simulink model "ACC_Model"  (Simulink 7.6)
settings: Solver=ode5  StartTime=0.0  StopTime=inf  FixedStep=1/100  RelTol=1e-3
undefined symbols (not defined in the file or in its folder): DiscIntNeverNeededParam
libraries: simulink x21, simulink_extras x6
(part 4 of 4)

== system ACC_Model/ACC_System/TIS2 ACC action/Stop & Go/If Action Subsystem/If Action Subsystem/If Action Subsystem1 ==
  e : Inport
  th_in : Inport  Port=2
  Action Port : ActionPort  PropagateVarSize=During execution  ActionType=else
  Constant : Constant  Value=0
  Constant1 : Constant  Value=0
  Rate Limiter : RateLimiter  RisingSlewLimit=BrakeMax*1e3  FallingSlewLimit=-BrakeMax*1e3  SampleTimeMode=inherited
  Saturation Dynamic : simulink/Discontinuities/Saturation Dynamic  SystemSampleTime=-1  OutMin=[]  OutMax=[]  OutDataTypeStr=Inherit: Same as second input  OutDataType=fixdt(1, 16)  OutScaling=2^-10  DoSatur=off
  Subsystem : Subsystem
  brake : Outport  InitialOutput=0
  throttle : Outport  Port=2  InitialOutput=0
  wires:
  Subsystem/1(out) -> Saturation Dynamic/2
  e/1 -> Subsystem/1(e)
  Saturation Dynamic/1 -> Rate Limiter/1
  Constant/1 -> brake/1
  Rate Limiter/1 -> throttle/1
  th_in/1 -> Saturation Dynamic/1
  Constant1/1 -> Saturation Dynamic/3

== system ACC_Model/ACC_System/TIS1 ACC action/If Action Subsystem/If Action Subsystem1/If Action Subsystem1/If Action Subsystem/Subsystem ==
  e : Inport
  Difference : simulink/Discrete/Difference  SystemSampleTime=-1  ICPrevInput=0.0  OutMin=[]  OutMax=[]  OutDataType=sfix(16)  OutScaling=2^-10  DoSatur=off
  Discrete-Time Integrator : DiscreteIntegrator  SampleTime=-1  ICPrevOutput=DiscIntNeverNeededParam  ICPrevScaledInput=DiscIntNeverNeededParam
  Gain : Gain  Gain=100
  Gain1 : Gain  Gain=0.3
  Gain2 : Gain  Gain=3.065*0.01
  Sum : Sum  Inputs=+++
  out : Outport
  wires:
  e/1 -> Gain1/1, Gain/1, Gain2/1
  Gain1/1 -> Discrete-Time Integrator/1
  Gain2/1 -> Difference/1
  Gain/1 -> Sum/1
  Discrete-Time Integrator/1 -> Sum/2
  Difference/1 -> Sum/3
  Sum/1 -> out/1

== system ACC_Model/ACC_System/TIS2 ACC action/If Action Subsystem/If Action Subsystem1/If Action Subsystem1/If Action Subsystem/Subsystem ==
  e : Inport
  Difference : simulink/Discrete/Difference  SystemSampleTime=-1  ICPrevInput=0.0  OutMin=[]  OutMax=[]  OutDataType=sfix(16)  OutScaling=2^-10  DoSatur=off
  Discrete-Time Integrator : DiscreteIntegrator  SampleTime=-1  ICPrevOutput=DiscIntNeverNeededParam  ICPrevScaledInput=DiscIntNeverNeededParam
  Gain : Gain  Gain=100
  Gain1 : Gain  Gain=0.3
  Gain2 : Gain  Gain=3.065*0.01
  Sum : Sum  Inputs=+++
  out : Outport
  wires:
  e/1 -> Gain1/1, Gain/1, Gain2/1
  Gain1/1 -> Discrete-Time Integrator/1
  Gain2/1 -> Difference/1
  Gain/1 -> Sum/1
  Discrete-Time Integrator/1 -> Sum/2
  Difference/1 -> Sum/3
  Sum/1 -> out/1

== system ACC_Model/ACC_System/TIS2 ACC action/Stop & Go/If Action Subsystem/If Action Subsystem/If Action Subsystem1/Subsystem ==
  e : Inport
  Difference : simulink/Discrete/Difference  SystemSampleTime=-1  ICPrevInput=0.0  OutMin=[]  OutMax=[]  OutDataType=sfix(16)  OutScaling=2^-10  DoSatur=off
  Discrete-Time Integrator : DiscreteIntegrator  SampleTime=-1  ICPrevOutput=DiscIntNeverNeededParam  ICPrevScaledInput=DiscIntNeverNeededParam
  Gain : Gain  Gain=20
  Gain1 : Gain  Gain=0.3
  Gain2 : Gain  Gain=3.065*0.01
  Sum : Sum  Inputs=+++
  out : Outport
  wires:
  e/1 -> Gain1/1, Gain/1, Gain2/1
  Gain1/1 -> Discrete-Time Integrator/1
  Gain2/1 -> Difference/1
  Gain/1 -> Sum/1
  Discrete-Time Integrator/1 -> Sum/2
  Difference/1 -> Sum/3
  Sum/1 -> out/1

== matlab function ACC_System/TIS1 Bend Road/Embedded MATLAB Function ==
  data: TISMaxRange parameter double; index output double; distance input double; TISdet parameter double
function index = clsst_bjct(TISMaxRange, distance, TISdet)
% which object is the closest?

[mini, index] = min(distance);
if mini == TISMaxRange(1)
    index = TISdet(1);
end
end

== matlab function ACC_System/TIS2 Bend Road/TIS2_closest_object_search1 ==
  data: TISMaxRange parameter double; distance input double; index output double; TISdet parameter double
function index = clsst_bjct(TISMaxRange, distance, TISdet)
% which object is the closest?

[mini, index] = min(distance);
if mini == 5*TISMaxRange(2)
    index = TISdet(2);
end
end

== matlab function ACC_System/TIS1 Straight Road/TIS1_closest_object_search ==
  data: distance input double; index output double; TISMaxRange parameter double; TISdet parameter double
function index = clsst_bjct(distance, TISMaxRange, TISdet)
% which object is the closest?

[mini, index] = min(distance);
if mini == TISMaxRange(1)
    index = TISdet(1);
end

end

== matlab function ACC_System/TIS2 Straight Road/TIS2_closest_object_search ==
  data: distance input double; index output double; TISMaxRange parameter double; TISdet parameter double
function index = clsst_bjct(distance, TISMaxRange, TISdet)
% which object is the closest?

[mini, index] = min(distance);
if mini == 5*TISMaxRange(2)
    index = TISdet(2);
end
end
